simulink library "SimplusGT"  (R2018b)
settings: Solver=ode45  StartTime=0.0  StopTime=10.0  RelTol=1e-3
undefined symbols (not defined in the file): ang_r, Cf, DiscIntNeverNeededParam, initial, Lc, Lf, m, OtherInputs, P_dc, Sbase, t0, Tm_pu, Ts, V, Vbase, w_droop, w_i, w_pll, w_tau, w_v, Wbase, wc, wfil, x0, Ybase, Zbase
libraries: powerlib x334, SimplexPS_2015a x6, $bdroot x1
(part 3 of 8)

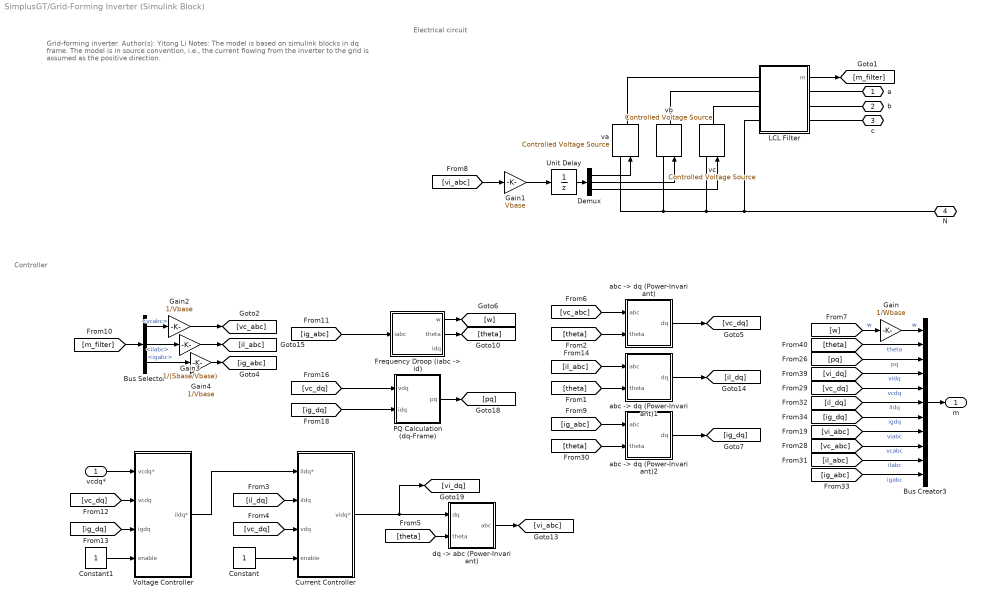
== system SimplusGT/Grid-Forming Inverter (Simulink Block) ==
  note: Controller
  note: Electrical circuit
  note: Grid-forming inverter.
      |
      | Author(s): Yitong Li
      |
      | Notes:
      |
      | The model is based on simulink blocks in dq frame.
      |
      | The model is in source convention, i.e., the current flowing from the inverter to the grid is assumed as the positive direction.
  vcdq* : Inport
  Bus Creator3 : BusCreator  Inputs=11
  Bus Selector : BusSelector  OutputSignals=vcabc,ilabc,igabc
  Constant : Constant
  Constant1 : Constant
  Current Controller : Subsystem  mask{Ts=Ts, Wbase=Wbase, Lf=Lf*(Vbase^2/Sbase)/Wbase, Kg=0, Kp=w_i*Lf*(Vbase^2/Sbase)/Wbase, Ki=w_i*w_i/4*Lf*(Vbase^2/Sbase)/Wbase, xdmax=inf, xqmax=inf, Kcd=0}
      mask prompts: Ts "Sampling Time (s)"; Wbase "Base Angular Frequency (rad/s)"; Lf "Inductance"; Kg "Estimator Gain"; Kp "Proportional Gain"; Ki "Integral Gain"; xdmax "Voltage D Limit"; xqmax "Voltage Q Limit"; Kcd "Cross Decoupling Gain"
  Demux : Demux  Outputs=3
  "Frequency Droop (iabc -> id)" : Subsystem  AncestorBlock=|  mask{Ts=Ts, Sbase=Sbase, Vbase=Vbase, Wbase=Wbase, m=m, w_tau=w_droop, theta0=0, i0=0, w0=1}
      | SimplusGT/Frequency Droop
      | (iabc -> id)
      mask prompts: Ts "Ts (s), samping period"; Sbase "Sbase (VA), base power"; Vbase "Vbase (V), base voltage"; Wbase "Wbase (rad/s), base angular frequency"; m "m (pu), droop gain"; w_tau "w_tau (rad/s), low-pass filter bandwidth"; theta0 "theta0 (rad), initial angle"; i0 "i0 (pu), current setting point"; w0 "w0 (pu), frequency setting point"
  Gain : Gain  Gain=1/Wbase
  Gain1 : Gain  Gain=Vbase
  Gain2 : Gain  Gain=1/Vbase
  Gain3 : Gain  Gain=1/(Sbase/Vbase)
  Gain4 : Gain  Gain=1/Vbase
  LCL Filter : Subsystem  AncestorBlock=SimplexPS/LCL Filter  mask{Lf=Lf*(Vbase^2/Sbase)/Wbase, Rf=1e-9, Lc=Lc*(Vbase^2/Sbase)/Wbase, Rc=1e-9, Cf=Cf*(Sbase/Vbase^2)/Wbase, Rd=1e-20}
      mask prompts: Lf "Lf (H)"; Rf "Rf (Ohm)"; Lc "Lc (H)"; Rc "Rc (Ohm)"; Cf "Cf (F)"; Rd "Rd (Ohm)"
  PQ Calculation (dq-Frame) : Subsystem  AncestorBlock=|
      | SimplusGT/PQ Calculation
      | (dq-Frame)
  Unit Delay : UnitDelay  SampleTime=-1
  Voltage Controller : Subsystem  mask{Ts=Ts, Wbase=Wbase, Cf=Cf*(Sbase/Vbase^2)/Wbase, Kg=0, Kp=w_v*Cf*(Sbase/Vbase^2)/Wbase, Ki=w_v*w_v/4*Cf*(Sbase/Vbase^2)/Wbase*100, xdmax=inf, xqmax=inf, Kcd=0}
      mask prompts: Ts "Sampling Time (s)"; Wbase "Base Angular Frequency (rad/s)"; Cf "Capacitance"; Kg "Estimator Gain"; Kp "Proportional Gain"; Ki "Integral Gain"; xdmax "Current D Limit"; xqmax "Current Q Limit"; Kcd "Cross Decoupling Gain"
  "abc -> dq (Power-Invariant)" : Subsystem  AncestorBlock=|
      | SimplusGT/abc -> dq
      | (Power-Invariant)
  "abc -> dq (Power-Invariant)1" : Subsystem  AncestorBlock=|
      | SimplusGT/abc -> dq
      | (Power-Invariant)
  "abc -> dq (Power-Invariant)2" : Subsystem  AncestorBlock=|
      | SimplusGT/abc -> dq
      | (Power-Invariant)
  "dq -> abc (Power-Invariant)" : Subsystem  AncestorBlock=|
      | SimplusGT/dq -> abc
      | (Power-Invariant)
  va : powerlib/Electrical Sources/Controlled Voltage Source  Initialize=on  Source_Type=AC  Amplitude=0  Phase=0  Frequency=0  Measurements=None
  vb : powerlib/Electrical Sources/Controlled Voltage Source  Initialize=on  Source_Type=AC  Amplitude=0  Phase=0  Frequency=0  Measurements=None
  vc : powerlib/Electrical Sources/Controlled Voltage Source  Initialize=on  Source_Type=AC  Amplitude=0  Phase=0  Frequency=0  Measurements=None
  a : PMIOPort  Side=Right
  b : PMIOPort  Port=2  Side=Right
  c : PMIOPort  Port=3  Side=Right
  N : PMIOPort  Port=4  Side=Right
  m : Outport
  wires:
  "dq -> abc (Power-Invariant)"/1(abc) -> [vi_abc]
  Bus Creator3/1 -> m/1
  LCL Filter/1(m) -> [m_filter]
  Demux/1 -> va/1
  Demux/2 -> vb/1
  Demux/3 -> vc/1
  [theta] -> "abc -> dq (Power-Invariant)"/2(theta)
  [theta] -> "abc -> dq (Power-Invariant)1"/2(theta)
  [vc_abc] -> "abc -> dq (Power-Invariant)"/1(abc)
  [il_abc] -> "abc -> dq (Power-Invariant)1"/1(abc)
  [ig_abc] -> "abc -> dq (Power-Invariant)2"/1(abc)
  [theta] -> "abc -> dq (Power-Invariant)2"/2(theta)
  Bus Selector/3 -> Gain4/1  "<igabc>"
  Bus Selector/2 -> Gain3/1  "<ilabc>"
  "Frequency Droop (iabc -> id)"/2(theta) -> [theta]
  "Frequency Droop (iabc -> id)"/1(w) -> [w]
  Constant/1 -> Current Controller/4(enable)
  [vc_dq] -> Current Controller/3(vdq)
  Current Controller/1(vidq*) -> [vi_dq], "dq -> abc (Power-Invariant)"/1(dq)
  [theta] -> "dq -> abc (Power-Invariant)"/2(theta)
  [vc_dq] -> PQ Calculation (dq-Frame)/1(vdq)
  PQ Calculation (dq-Frame)/1(pq) -> [pq]
  [ig_dq] -> PQ Calculation (dq-Frame)/2(idq)
  [il_dq] -> Current Controller/2(iIdq)
  [ig_abc] -> "Frequency Droop (iabc -> id)"/1(iabc)
  "abc -> dq (Power-Invariant)"/1(dq) -> [vc_dq]
  "abc -> dq (Power-Invariant)2"/1(dq) -> [ig_dq]
  "abc -> dq (Power-Invariant)1"/1(dq) -> [il_dq]
  [m_filter] -> Bus Selector/1
  Unit Delay/1 -> Demux/1
  Bus Selector/1 -> Gain2/1  "<vcabc>"
  [w] -> Gain/1  "w"
  Gain/1 -> Bus Creator3/1  "w"
  [theta] -> Bus Creator3/2  "theta"
  [pq] -> Bus Creator3/3  "pq"
  [vi_dq] -> Bus Creator3/4  "vidq"
  [vc_dq] -> Bus Creator3/5  "vcdq"
  [il_dq] -> Bus Creator3/6  "ildq"
  [ig_dq] -> Bus Creator3/7  "igdq"
  [vi_abc] -> Bus Creator3/8  "viabc"
  [vc_abc] -> Bus Creator3/9  "vcabc"
  [il_abc] -> Bus Creator3/10  "ilabc"
  [ig_abc] -> Bus Creator3/11  "igabc"
  vcdq*/1 -> Voltage Controller/1(vcdq*)
  Voltage Controller/1(ildq*) -> Current Controller/1(iIdq*)
  Constant1/1 -> Voltage Controller/4(enable)
  [vc_dq] -> Voltage Controller/2(vcdq)
  [ig_dq] -> Voltage Controller/3(igdq)
  Gain2/1 -> [vc_abc]
  Gain3/1 -> [il_abc]
  Gain4/1 -> [ig_abc]
  [vi_abc] -> Gain1/1
  Gain1/1 -> Unit Delay/1
  connections:
  LCL Filter/LConn2 -- vb/RConn1
  LCL Filter/LConn1 -- va/RConn1
  LCL Filter/RConn1 -- a/RConn1
  LCL Filter/RConn2 -- b/RConn1
  LCL Filter/RConn3 -- c/RConn1
  N/RConn1 -- LCL Filter/LConn4 -- vc/LConn1 -- vb/LConn1 -- va/LConn1
  LCL Filter/LConn3 -- vc/RConn1

== system SimplusGT/Hold ==
  note: Hold
      |
      | Author(s): Yitong Li
      |
      | Notes:
      |
      | This block can hold the input value to constant when "enable" is set from zero to one.
  In : Inport
  Enable : Inport  Port=2
  Memory : Memory
  Switch : Switch  Criteria=u2 > Threshold  Threshold=0.5
  Out : Outport
  wires:
  Switch/1 -> Memory/1, Out/1
  Enable/1 -> Switch/2
  Memory/1 -> Switch/1
  In/1 -> Switch/3

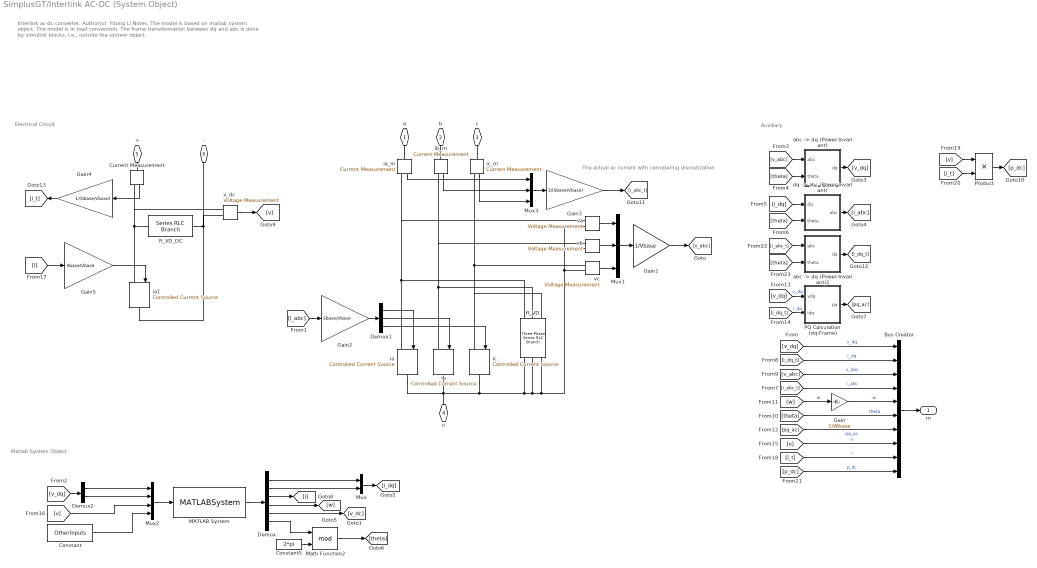
== system SimplusGT/Interlink AC-DC (System Object) ==
  note: Matlab System Object
  note: Auxiliary
  note: Electrical Circuit
  note: Interlink ac-dc converter.
      |
      | Author(s): Yitong Li
      |
      | Notes:
      |
      | The model is based on matlab system object.
      |
      | The model is in load convention.
      |
      | The frame transformation between dq and abc is done by simulink blocks, i.e., outside the system object.
  note: The actual ac current with considering discretization
  Bus Creator : BusCreator  Inputs=10
  Constant : Constant  Value=OtherInputs
  Constant5 : Constant  Value=2*pi
  Current Measurement : powerlib/Measurements/Current Measurement  PhasorSimulation=off  OutputType=Complex  PSBequivalent=0
  Demux : Demux  Outputs=6
  Demux1 : Demux  Outputs=3
  Demux2 : Demux  Outputs=2
  Gain : Gain  Gain=1/Wbase
  Gain1 : Gain  Gain=1/Vbase
  Gain2 : Gain  Gain=Sbase/Vbase
  Gain3 : Gain  Gain=1/(Sbase/Vbase)
  Gain4 : Gain  Gain=1/(Sbase/Vbase)
  Gain5 : Gain  Gain=Sbase/Vbase
  MATLAB System : MATLABSystem  System=SimplusGT.Class.InterlinkAcDc  Ts=Ts  Para=ApparatusPara  ApparatusType=ApparatusType  PowerFlow=PowerFlow  x0=x0  DiscreMethod=DiscreMethod  LinearizationTimes=LinearizationTimes  DirectFeedthrough=DirectFeedthrough  VirtualResistor=DiscreDampingFlag  EquiInitial=true  ElecPortIOs=[ 1, 2, 3 ]  SimulateUsing=Code generation
      mask Type: SimplusGT.Class.InterlinkAcDc
      mask Display:
      | disp('InterlinkAcDc');
      | port_label('input',1,'u');
      | port_label('output',1,'y');
  Math Function2 : Math  Operator=mod  SaturateOnIntegerOverflow=on
  Mux : Mux  Inputs=2
  Mux1 : Mux  Inputs=3
  Mux2 : Mux
  Mux3 : Mux  Inputs=3
  PQ Calculation (dq-Frame) : Subsystem  AncestorBlock=|
      | SimplusGT/PQ Calculation
      | (dq-Frame)
  Product : Product
  R_VD : powerlib/Elements/Three-Phase Series RLC Branch  LConnTagsString=A|B|C  RConnTagsString=A|B|C  BranchType=R  Resistance=DiscreDampingValue*Vbase^2/Sbase  Inductance=1e-3  Capacitance=1e-6  Measurements=None
  R_VD_DC : powerlib/Elements/Series RLC Branch  LConnTagsString=__new0  RConnTagsString=__new0  BranchType=R  Resistance=DiscreDampingValue*Vbase^2/Sbase  Inductance=1e-3  SetiL0=off  InitialCurrent=0  Capacitance=1e-6  Setx0=off  InitialVoltage=0  Measurements=None
  "abc -> dq (Power-Invariant)" : Subsystem  AncestorBlock=|
      | SimplusGT/abc -> dq
      | (Power-Invariant)
  "abc -> dq (Power-Invariant)1" : Subsystem  AncestorBlock=|
      | SimplusGT/abc -> dq
      | (Power-Invariant)
  "dq -> abc (Power-Invariant)" : Subsystem  AncestorBlock=|
      | SimplusGT/dq -> abc
      | (Power-Invariant)
  ia : powerlib/Electrical Sources/Controlled Current Source  Initialize=on  Source_Type=AC  Amplitude=0  Phase=0  Frequency=0  Measurements=None
  ia1 : powerlib/Electrical Sources/Controlled Current Source  Initialize=on  Source_Type=AC  Amplitude=0  Phase=0  Frequency=0  Measurements=None
  ia_m : powerlib/Measurements/Current Measurement  PhasorSimulation=off  OutputType=Complex  PSBequivalent=0
  ib : powerlib/Electrical Sources/Controlled Current Source  Initialize=on  Source_Type=AC  Amplitude=0  Phase=0  Frequency=0  Measurements=None
  ib_m : powerlib/Measurements/Current Measurement  PhasorSimulation=off  OutputType=Complex  PSBequivalent=0
  ic : powerlib/Electrical Sources/Controlled Current Source  Initialize=on  Source_Type=AC  Amplitude=0  Phase=0  Frequency=0  Measurements=None
  ic_m : powerlib/Measurements/Current Measurement  PhasorSimulation=off  OutputType=Complex  PSBequivalent=0
  v_dc : powerlib/Measurements/Voltage Measurement  PhasorSimulation=off  OutputType=Complex  PSBequivalent=0
  va : powerlib/Measurements/Voltage Measurement  PhasorSimulation=off  OutputType=Complex  PSBequivalent=0
  vb : powerlib/Measurements/Voltage Measurement  PhasorSimulation=off  OutputType=Complex  PSBequivalent=0
  vc : powerlib/Measurements/Voltage Measurement  PhasorSimulation=off  OutputType=Complex  PSBequivalent=0
  a : PMIOPort  Side=Left
  b : PMIOPort  Port=2  Side=Left
  c : PMIOPort  Port=3  Side=Left
  n : PMIOPort  Port=4  Side=Left
  + : PMIOPort  Port=5  Side=Left
  - : PMIOPort  Port=6  Side=Left
  m : Outport
  wires:
  Demux/2 -> Mux/2
  Demux/1 -> Mux/1
  Mux/1 -> [i_dq]
  Demux1/1 -> ia/1
  Demux1/2 -> ib/1
  va/1 -> Mux1/1
  vb/1 -> Mux1/2
  Mux1/1 -> Gain1/1
  [v_dq] -> Demux2/1
  Demux2/1 -> Mux2/1
  Demux2/2 -> Mux2/2
  [v_dq] -> Bus Creator/1  "v_dq"
  [i_dq_t] -> Bus Creator/2  "i_dq"
  [v_abc] -> Bus Creator/3  "v_abc"
  [i_abc_t] -> Bus Creator/4  "i_abc"
  [theta] -> Bus Creator/6  "theta"
  [v_abc] -> "abc -> dq (Power-Invariant)"/1(abc)
  [theta] -> "abc -> dq (Power-Invariant)"/2(theta)
  "abc -> dq (Power-Invariant)"/1(dq) -> [v_dq]
  [i_dq] -> "dq -> abc (Power-Invariant)"/1(dq)
  [theta] -> "dq -> abc (Power-Invariant)"/2(theta)
  "dq -> abc (Power-Invariant)"/1(abc) -> [i_abc]
  Mux2/1 -> MATLAB System/1
  MATLAB System/1 -> Demux/1
  vc/1 -> Mux1/3
  Demux1/3 -> ic/1
  Constant5/1 -> Math Function2/2
  Math Function2/1 -> [theta]
  Bus Creator/1 -> m/1
  Constant/1 -> Mux2/4
  [w] -> Gain/1  "w"
  Gain/1 -> Bus Creator/5  "w"
  [i_abc] -> Gain2/1
  [pq_ac] -> Bus Creator/7  "pq_ac"
  [v_dq] -> PQ Calculation (dq-Frame)/1(vdq)  "v_dq"
  [i_dq_t] -> PQ Calculation (dq-Frame)/2(idq)  "i_dq"
  PQ Calculation (dq-Frame)/1(pq) -> [pq_ac]
  Gain2/1 -> Demux1/1
  Gain1/1 -> [v_abc]
  [v] -> Bus Creator/8  "v"
  Demux/4 -> [w]
  Demux/5 -> [v_dc]
  Demux/6 -> Math Function2/1
  [v] -> Mux2/3
  Demux/3 -> [i]
  v_dc/1 -> [v]
  [i_t] -> Bus Creator/9  "i"
  [v] -> Product/1
  [i_t] -> Product/2
  Product/1 -> [p_dc]
  [p_dc] -> Bus Creator/10  "p_dc"
  ic_m/1 -> Mux3/3
  ib_m/1 -> Mux3/2
  Gain3/1 -> [i_abc_t]
  Mux3/1 -> Gain3/1
  ia_m/1 -> Mux3/1
  [theta] -> "abc -> dq (Power-Invariant)1"/2(theta)
  [i_abc_t] -> "abc -> dq (Power-Invariant)1"/1(abc)
  "abc -> dq (Power-Invariant)1"/1(dq) -> [i_dq_t]
  Gain4/1 -> [i_t]
  Current Measurement/1 -> Gain4/1
  [i] -> Gain5/1
  Gain5/1 -> ia1/1
  connections:
  vb/LConn2 -- va/LConn2 -- vc/LConn2 -- R_VD/RConn3 -- R_VD/RConn2 -- R_VD/RConn1 -- ic/RConn1 -- ia/RConn1 -- ib/RConn1 -- n/RConn1
  R_VD/LConn1 -- ia_m/RConn1 -- va/LConn1 -- ia/LConn1
  R_VD/LConn2 -- ib_m/RConn1 -- vb/LConn1 -- ib/LConn1
  R_VD/LConn3 -- ic/LConn1 -- ic_m/RConn1 -- vc/LConn1
  ia1/LConn1 -- Current Measurement/RConn1 -- v_dc/LConn1 -- R_VD_DC/LConn1
  ia1/RConn1 -- R_VD_DC/RConn1 -- -/RConn1 -- v_dc/LConn2
  c/RConn1 -- ic_m/LConn1
  b/RConn1 -- ib_m/LConn1
  a/RConn1 -- ia_m/LConn1
  Current Measurement/LConn1 -- +/RConn1

== system SimplusGT/L Filter (3ph) ==
  note: Model for a L filter.
      |
      | Author(s): Yitong Li
      |
      | Notes:
      |
      | vi is the converter side voltage, and vg is the grid side voltage.
  Bus Creator : BusCreator  Inputs=3
  "LL -> LN" : Subsystem  AncestorBlock=SimplusGT/LL -> LN
  "LL -> LN1" : Subsystem  AncestorBlock=SimplusGT/LL -> LN
  Mux : Mux  Inputs=3
  Mux1 : Mux  Inputs=3
  Mux2 : Mux  Inputs=3
  Three-Phase Series RLC Branch : powerlib/Elements/Three-Phase Series RLC Branch  LConnTagsString=A|B|C  RConnTagsString=A|B|C  BranchType=RL  Resistance=Rf  Inductance=Lf  Capacitance=1e-6  Measurements=None
  Vab : powerlib/Measurements/Voltage Measurement  PhasorSimulation=off  OutputType=Complex  PSBequivalent=0
  Vab1 : powerlib/Measurements/Voltage Measurement  PhasorSimulation=off  OutputType=Complex  PSBequivalent=0
  Vbc : powerlib/Measurements/Voltage Measurement  PhasorSimulation=off  OutputType=Complex  PSBequivalent=0
  Vbc1 : powerlib/Measurements/Voltage Measurement  PhasorSimulation=off  OutputType=Complex  PSBequivalent=0
  Vca : powerlib/Measurements/Voltage Measurement  PhasorSimulation=off  OutputType=Complex  PSBequivalent=0
  Vca1 : powerlib/Measurements/Voltage Measurement  PhasorSimulation=off  OutputType=Complex  PSBequivalent=0
  ila : powerlib/Measurements/Current Measurement  PhasorSimulation=off  OutputType=Complex  PSBequivalent=0
  ilb : powerlib/Measurements/Current Measurement  PhasorSimulation=off  OutputType=Complex  PSBequivalent=0
  ilc : powerlib/Measurements/Current Measurement  PhasorSimulation=off  OutputType=Complex  PSBequivalent=0
  via : PMIOPort  Side=Left
  vib : PMIOPort  Port=2  Side=Left
  vic : PMIOPort  Port=3  Side=Left
  vga : PMIOPort  Port=4  Side=Right
  vgb : PMIOPort  Port=5  Side=Right
  vgc : PMIOPort  Port=6  Side=Right
  m : Outport
  wires:
  Vab/1 -> Mux/1
  Vbc/1 -> Mux/2
  ilb/1 -> Mux2/2
  Vca/1 -> Mux/3
  Vca1/1 -> Mux1/3
  "LL -> LN1"/1(Out1) -> [vgabc]
  ilc/1 -> Mux2/3
  "LL -> LN"/1(Out1) -> [viabc]
  Mux1/1 -> "LL -> LN"/1(In1)
  Mux/1 -> "LL -> LN1"/1(In1)
  Vab1/1 -> Mux1/1
  ila/1 -> Mux2/1
  Mux2/1 -> [ilabc]
  Vbc1/1 -> Mux1/2
  [viabc] -> Bus Creator/1  "viabc"
  Bus Creator/1 -> m/1
  [vgabc] -> Bus Creator/2  "vgabc"
  [ilabc] -> Bus Creator/3  "ilabc"
  connections:
  Vca/LConn1 -- Vbc/LConn2 -- ilc/RConn1 -- vgc/RConn1
  Three-Phase Series RLC Branch/LConn1 -- via/RConn1 -- Vab1/LConn1 -- Vca1/LConn2
  Three-Phase Series RLC Branch/RConn2 -- ilb/LConn1
  Three-Phase Series RLC Branch/RConn3 -- ilc/LConn1
  Vab/LConn2 -- Vbc/LConn1 -- vgb/RConn1 -- ilb/RConn1
  Vbc1/LConn2 -- vic/RConn1 -- Three-Phase Series RLC Branch/LConn3 -- Vca1/LConn1
  Vab1/LConn2 -- vib/RConn1 -- Three-Phase Series RLC Branch/LConn2 -- Vbc1/LConn1
  Vca/LConn2 -- Vab/LConn1 -- ila/RConn1 -- vga/RConn1
  Three-Phase Series RLC Branch/RConn1 -- ila/LConn1

== system SimplusGT/LC Filter (3ph) ==
  note: Model for a LC filter.
      |
      | Author(s): Yitong Li
      |
      | Notes:
      |
      | vi is the converter side voltage, and vg is the grid side voltage.
  Bus Creator : BusCreator  Inputs=4
  "LL -> LN" : Subsystem  AncestorBlock=SimplusGT/LL -> LN
  Mux{1..4} (4 alike) : Mux  Inputs=3
  Three-Phase Series RLC Branch : powerlib/Elements/Three-Phase Series RLC Branch  LConnTagsString=A|B|C  RConnTagsString=A|B|C  BranchType=RL  Resistance=Rf  Inductance=Lf  Capacitance=1e-6  Measurements=None
  Three-Phase Series RLC Branch2 : powerlib/Elements/Three-Phase Series RLC Branch  LConnTagsString=A|B|C  RConnTagsString=A|B|C  BranchType=RC  Resistance=Rd  Inductance=Lc  Capacitance=Cf  Measurements=None
  Vab1 : powerlib/Measurements/Voltage Measurement  PhasorSimulation=off  OutputType=Complex  PSBequivalent=0
  Vbc1 : powerlib/Measurements/Voltage Measurement  PhasorSimulation=off  OutputType=Complex  PSBequivalent=0
  Vca1 : powerlib/Measurements/Voltage Measurement  PhasorSimulation=off  OutputType=Complex  PSBequivalent=0
  iga : powerlib/Measurements/Current Measurement  PhasorSimulation=off  OutputType=Complex  PSBequivalent=0
  igb : powerlib/Measurements/Current Measurement  PhasorSimulation=off  OutputType=Complex  PSBequivalent=0
  igc : powerlib/Measurements/Current Measurement  PhasorSimulation=off  OutputType=Complex  PSBequivalent=0
  ila : powerlib/Measurements/Current Measurement  PhasorSimulation=off  OutputType=Complex  PSBequivalent=0
  ilb : powerlib/Measurements/Current Measurement  PhasorSimulation=off  OutputType=Complex  PSBequivalent=0
  ilc : powerlib/Measurements/Current Measurement  PhasorSimulation=off  OutputType=Complex  PSBequivalent=0
  vca measure : powerlib/Measurements/Voltage Measurement  PhasorSimulation=off  OutputType=Complex  PSBequivalent=0
  vcb measure : powerlib/Measurements/Voltage Measurement  PhasorSimulation=off  OutputType=Complex  PSBequivalent=0
  vcc measure : powerlib/Measurements/Voltage Measurement  PhasorSimulation=off  OutputType=Complex  PSBequivalent=0
  via : PMIOPort  Side=Left
  vib : PMIOPort  Port=2  Side=Left
  vic : PMIOPort  Port=3  Side=Left
  vga : PMIOPort  Port=4  Side=Right
  vgb : PMIOPort  Port=5  Side=Right
  vgc : PMIOPort  Port=6  Side=Right
  N : PMIOPort  Port=7  Side=Left
  m : Outport
  wires:
  igb/1 -> Mux4/2
  iga/1 -> Mux4/1
  Vab1/1 -> Mux1/1
  vcb measure/1 -> Mux3/2
  [viabc] -> Bus Creator/1  "viabc"
  ilc/1 -> Mux2/3
  igc/1 -> Mux4/3
  ila/1 -> Mux2/1
  Mux1/1 -> "LL -> LN"/1(In1)
  Bus Creator/1 -> m/1
  vcc measure/1 -> Mux3/3
  ilb/1 -> Mux2/2
  vca measure/1 -> Mux3/1
  Mux3/1 -> [vcabc]
  "LL -> LN"/1(Out1) -> [viabc]
  Vca1/1 -> Mux1/3
  [vcabc] -> Bus Creator/2  "vcabc"
  Mux2/1 -> [ilabc]
  Mux4/1 -> [igabc]
  Vbc1/1 -> Mux1/2
  [ilabc] -> Bus Creator/3  "ilabc"
  [igabc] -> Bus Creator/4  "igabc"
  connections:
  Three-Phase Series RLC Branch2/LConn3 -- igc/LConn1 -- ilc/RConn1 -- vcc measure/LConn1
  Vbc1/LConn2 -- vic/RConn1 -- Three-Phase Series RLC Branch/LConn3 -- Vca1/LConn1
  Three-Phase Series RLC Branch/RConn3 -- ilc/LConn1
  vca measure/LConn1 -- ila/RConn1 -- iga/LConn1 -- Three-Phase Series RLC Branch2/LConn1
  vga/RConn1 -- iga/RConn1
  vgb/RConn1 -- igb/RConn1
  vcb measure/LConn1 -- igb/LConn1 -- ilb/RConn1 -- Three-Phase Series RLC Branch2/LConn2
  Vab1/LConn2 -- vib/RConn1 -- Three-Phase Series RLC Branch/LConn2 -- Vbc1/LConn1
  vgc/RConn1 -- igc/RConn1
  vcc measure/LConn2 -- vca measure/LConn2 -- vcb measure/LConn2 -- N/RConn1 -- Three-Phase Series RLC Branch2/RConn1 -- Three-Phase Series RLC Branch2/RConn2 -- Three-Phase Series RLC Branch2/RConn3
  Three-Phase Series RLC Branch/LConn1 -- via/RConn1 -- Vab1/LConn1 -- Vca1/LConn2
  Three-Phase Series RLC Branch/RConn1 -- ila/LConn1
  Three-Phase Series RLC Branch/RConn2 -- ilb/LConn1

== system SimplusGT/LCL Filter (3ph) ==
  note: Model for a LCL filter.
      |
      | Author(s): Yitong Li
      |
      | Notes:
      |
      | vi is the converter side voltage, and vg is the grid side voltage.
  Bus Creator : BusCreator  Inputs=5
  "LL -> LN" : SimplexPS_2015a/LL -> LN  SystemSampleTime=-1
      settings: SourceProductName=Some kind of I/O error occurred when accessing database \\icnas1.cc.ic.ac.uk\yz34218\appdata\MathWorks\MATLAB\R2018b\slblocks_master.db. (disk I/O error)
  "LL -> LN1" : SimplexPS_2015a/LL -> LN  SystemSampleTime=-1
      settings: SourceProductName=Some kind of I/O error occurred when accessing database \\icnas1.cc.ic.ac.uk\yz34218\appdata\MathWorks\MATLAB\R2018b\slblocks_master.db. (disk I/O error)
  Mux{,1..4} (5 alike) : Mux  Inputs=3
  Three-Phase Series RLC Branch : powerlib/Elements/Three-Phase Series RLC Branch  LConnTagsString=A|B|C  RConnTagsString=A|B|C  BranchType=RL  Resistance=Rf  Inductance=Lf  Capacitance=1e-6  Measurements=None
  Three-Phase Series RLC Branch1 : powerlib/Elements/Three-Phase Series RLC Branch  LConnTagsString=A|B|C  RConnTagsString=A|B|C  BranchType=RL  Resistance=Rc  Inductance=Lc  Capacitance=1e-6  Measurements=None
  Three-Phase Series RLC Branch2 : powerlib/Elements/Three-Phase Series RLC Branch  LConnTagsString=A|B|C  RConnTagsString=A|B|C  BranchType=RC  Resistance=Rd  Inductance=Lc  Capacitance=Cf  Measurements=None
  Vab : powerlib/Measurements/Voltage Measurement  PhasorSimulation=off  OutputType=Complex  PSBequivalent=0
  Vab1 : powerlib/Measurements/Voltage Measurement  PhasorSimulation=off  OutputType=Complex  PSBequivalent=0
  Vbc : powerlib/Measurements/Voltage Measurement  PhasorSimulation=off  OutputType=Complex  PSBequivalent=0
  Vbc1 : powerlib/Measurements/Voltage Measurement  PhasorSimulation=off  OutputType=Complex  PSBequivalent=0
  Vca : powerlib/Measurements/Voltage Measurement  PhasorSimulation=off  OutputType=Complex  PSBequivalent=0
  Vca1 : powerlib/Measurements/Voltage Measurement  PhasorSimulation=off  OutputType=Complex  PSBequivalent=0
  iga : powerlib/Measurements/Current Measurement  PhasorSimulation=off  OutputType=Complex  PSBequivalent=0
  igb : powerlib/Measurements/Current Measurement  PhasorSimulation=off  OutputType=Complex  PSBequivalent=0
  igc : powerlib/Measurements/Current Measurement  PhasorSimulation=off  OutputType=Complex  PSBequivalent=0
  ila : powerlib/Measurements/Current Measurement  PhasorSimulation=off  OutputType=Complex  PSBequivalent=0
  ilb : powerlib/Measurements/Current Measurement  PhasorSimulation=off  OutputType=Complex  PSBequivalent=0
  ilc : powerlib/Measurements/Current Measurement  PhasorSimulation=off  OutputType=Complex  PSBequivalent=0
  vca measure : powerlib/Measurements/Voltage Measurement  PhasorSimulation=off  OutputType=Complex  PSBequivalent=0
  vcb measure : powerlib/Measurements/Voltage Measurement  PhasorSimulation=off  OutputType=Complex  PSBequivalent=0
  vcc measure : powerlib/Measurements/Voltage Measurement  PhasorSimulation=off  OutputType=Complex  PSBequivalent=0
  via : PMIOPort  Side=Left
  vib : PMIOPort  Port=2  Side=Left
  vic : PMIOPort  Port=3  Side=Left
  vga : PMIOPort  Port=4  Side=Right
  vgb : PMIOPort  Port=5  Side=Right
  vgc : PMIOPort  Port=6  Side=Right
  N : PMIOPort  Port=7  Side=Left
  m : Outport
  wires:
  Mux4/1 -> [igabc]
  ilb/1 -> Mux2/2
  ila/1 -> Mux2/1
  igc/1 -> Mux4/3
  vcc measure/1 -> Mux3/3
  Vab/1 -> Mux/1
  Mux/1 -> "LL -> LN1"/1
  vca measure/1 -> Mux3/1
  vcb measure/1 -> Mux3/2
  igb/1 -> Mux4/2
  iga/1 -> Mux4/1
  Vca/1 -> Mux/3
  ilc/1 -> Mux2/3
  Vbc/1 -> Mux/2
  Mux2/1 -> [ilabc]
  Bus Creator/1 -> m/1
  "LL -> LN1"/1 -> [vgabc]
  Mux3/1 -> [vcabc]
  Vbc1/1 -> Mux1/2
  Vca1/1 -> Mux1/3
  Mux1/1 -> "LL -> LN"/1
  Vab1/1 -> Mux1/1
  "LL -> LN"/1 -> [viabc]
  [viabc] -> Bus Creator/1  "viabc"
  [vcabc] -> Bus Creator/2  "vcabc"
  [vgabc] -> Bus Creator/3  "vgabc"
  [ilabc] -> Bus Creator/4  "ilabc"
  [igabc] -> Bus Creator/5  "igabc"
  connections:
  vca measure/LConn2 -- Three-Phase Series RLC Branch2/RConn1 -- Three-Phase Series RLC Branch2/RConn2 -- N/RConn1 -- Three-Phase Series RLC Branch2/RConn3 -- vcc measure/LConn2 -- vcb measure/LConn2
  igc/RConn1 -- Vca/LConn1 -- Vbc/LConn2 -- vgc/RConn1
  Vbc1/LConn2 -- Three-Phase Series RLC Branch/LConn3 -- vic/RConn1 -- Vca1/LConn1
  Vab1/LConn2 -- vib/RConn1 -- Three-Phase Series RLC Branch/LConn2 -- Vbc1/LConn1
  Vca1/LConn2 -- Three-Phase Series RLC Branch/LConn1 -- via/RConn1 -- Vab1/LConn1
  ilc/RConn1 -- Three-Phase Series RLC Branch1/LConn3 -- vcc measure/LConn1 -- Three-Phase Series RLC Branch2/LConn3
  Three-Phase Series RLC Branch1/RConn2 -- igb/LConn1
  igb/RConn1 -- vgb/RConn1 -- Vbc/LConn1 -- Vab/LConn2
  vcb measure/LConn1 -- ilb/RConn1 -- Three-Phase Series RLC Branch1/LConn2 -- Three-Phase Series RLC Branch2/LConn2
  vca measure/LConn1 -- ila/RConn1 -- Three-Phase Series RLC Branch1/LConn1 -- Three-Phase Series RLC Branch2/LConn1
  Vca/LConn2 -- Vab/LConn1 -- vga/RConn1 -- iga/RConn1
  Three-Phase Series RLC Branch1/RConn1 -- iga/LConn1
  Three-Phase Series RLC Branch1/RConn3 -- igc/LConn1
  Three-Phase Series RLC Branch/RConn1 -- ila/LConn1
  Three-Phase Series RLC Branch/RConn2 -- ilb/LConn1
  Three-Phase Series RLC Branch/RConn3 -- ilc/LConn1

== system SimplusGT/LL -> LN ==
  note: Transformation from line-to-line voltage to line-to-neutral voltage.
      |
      | Author(s): Yitong Li
  In1 : Inport
  Fcn : Fcn  Expr=u[1]-u[3]
  Fcn1 : Fcn  Expr=u[2]-u[1]
  Fcn2 : Fcn  Expr=u[3]-u[2]
  Gain : Gain  Gain=1/3
  Mux9 : Mux  Inputs=3
  Out1 : Outport
  wires:
  Fcn/1 -> Mux9/1
  Fcn1/1 -> Mux9/2
  Fcn2/1 -> Mux9/3
  Mux9/1 -> Out1/1
  Gain/1 -> Fcn2/1, Fcn1/1, Fcn/1
  In1/1 -> Gain/1

== system SimplusGT/Load Impulse ==
  note: Model for an impulse load.
      |
      | Author(s): Yitong Li
  Single Pulse : $bdroot/Single Pulse  t0=t0  dt=dt  Am=1
  Three-Phase Breaker : powerlib/Elements/Three-Phase Breaker  InitialState=open  SwitchA=on  SwitchB=on  SwitchC=on  SwitchTimes="[1/60  5/60]"  External=on  BreakerResistance=0.01  SnubberResistance=1e6  SnubberCapacitance=inf  Measurements=None
  load : powerlib/Elements/Three-Phase Parallel RLC Branch  LConnTagsString=A|B|C  RConnTagsString=A|B|C  BranchType=R  Resistance=R  Inductance=1  Capacitance=1  Measurements=None
      settings: SourceProductName=Simscape Power Systems  SourceProductBaseCode=PS
  a : PMIOPort  Side=Left
  b : PMIOPort  Port=2  Side=Left
  c : PMIOPort  Port=3  Side=Left
  n : PMIOPort  Port=4  Side=Right
  wires:
  Single Pulse/1 -> Three-Phase Breaker/1
  connections:
  load/RConn2 -- load/RConn3 -- load/RConn1 -- n/RConn1
  Three-Phase Breaker/RConn1 -- load/LConn3
  Three-Phase Breaker/RConn2 -- load/LConn2
  Three-Phase Breaker/RConn3 -- load/LConn1
  c/RConn1 -- Three-Phase Breaker/LConn1
  b/RConn1 -- Three-Phase Breaker/LConn2
  a/RConn1 -- Three-Phase Breaker/LConn3

== system SimplusGT/Load Step ==
  note: Model for a step load.
      |
      | Author(s): Yitong Li
  Constant : Constant  Value=Reverse
  Step : Step  Time=t0  SampleTime=0
  Step1 : Step  Time=t0  Before=1  After=0  SampleTime=0
  Switch : Switch  Criteria=u2 > Threshold  Threshold=0.5
  Three-Phase Breaker : powerlib/Elements/Three-Phase Breaker  InitialState=open  SwitchA=on  SwitchB=on  SwitchC=on  SwitchTimes="[1/60  5/60]"  External=on  BreakerResistance=0.01  SnubberResistance=1e6  SnubberCapacitance=inf  Measurements=None
  load : powerlib/Elements/Three-Phase Parallel RLC Branch  LConnTagsString=A|B|C  RConnTagsString=A|B|C  BranchType=R  Resistance=R  Inductance=1  Capacitance=1  Measurements=None
      settings: SourceProductName=Simscape Power Systems  SourceProductBaseCode=PS
  a : PMIOPort  Side=Left
  b : PMIOPort  Port=2  Side=Left
  c : PMIOPort  Port=3  Side=Left
  n : PMIOPort  Port=4  Side=Right
  wires:
  Switch/1 -> Three-Phase Breaker/1
  Constant/1 -> Switch/2
  Step1/1 -> Switch/1
  Step/1 -> Switch/3
  connections:
  a/RConn1 -- Three-Phase Breaker/LConn3
  b/RConn1 -- Three-Phase Breaker/LConn2
  Three-Phase Breaker/RConn3 -- load/LConn1
  Three-Phase Breaker/RConn2 -- load/LConn2
  load/RConn2 -- n/RConn1 -- load/RConn3 -- load/RConn1
  Three-Phase Breaker/RConn1 -- load/LConn3
  c/RConn1 -- Three-Phase Breaker/LConn1

== system SimplusGT/PLL (vDQ -> vq) ==
  note: Gpll
  note: Measurement
  note: Phase lock loop (PLL)
      |
      | Author(s): Yitong Li
      |
      | Notes:
      |
      | vq is fed into the PI controller of the PLL.
      |
      | This PLL assumes the input voltage is in DQ frame, which is the common electrical frame. It is not a practical PLL which uses vabc as the input. But this PLL is useful in research.
  vDQ : Inport
  wDQ : Inport  Port=2
  Constant1 : Constant
  Constant2 : Constant  Value=theta0
  Constant3 : Constant
  Constant4 : Constant  Value=2*pi
  Constant6 : Constant  Value=0
  Demux1 : Demux  Outputs=2
  Discrete PI1 : Subsystem  AncestorBlock=SimplusGT/Discrete PI  mask{Kp=w_pll, Ki=w_pll*w_pll/4, xmax=inf, xmin=-inf, Ts=Ts}
      mask prompts: Kp "Proportional Gain"; Ki "Integral Gain"; xmax "Upper Limit"; xmin "Lower Limit"; Ts "Sampling Time"
  Discrete-Time Integrator : DiscreteIntegrator  SampleTime=Ts  ICPrevOutput=DiscIntNeverNeededParam  ICPrevScaledInput=DiscIntNeverNeededParam
  Filter p : DiscreteTransferFcn  Numerator=w_tau*Ts  Denominator=[1 ((w_tau*Ts)-1)]  SampleTime=Ts
  Gain1 : Gain  Gain=Wbase
  Gain2 : Gain  Gain=1/Vbase
  Gain4 : Gain  Gain=1/Wbase
  Gain5 : Gain  Gain=1/pi
  Math Function1 : Math  Operator=mod  SaturateOnIntegerOverflow=on
  Mux : Mux  Inputs=2
  Scope : Scope  NumInputPorts=4
  Sum : Sum
  Sum1 : Sum
  Sum2 : Sum  Inputs=+-
  "x1y1 -> x2y2" : Subsystem  AncestorBlock=SimplusGT/x1y1 -> x2y2
  wdq : Outport
  theta : Outport  Port=2
  vdq : Outport  Port=3
  wires:
  [theta0] -> Mux/1  "theta0"
  Constant2/1 -> [theta0], Sum1/2
  Math Function1/1 -> "x1y1 -> x2y2"/2(theta), theta/1, [theta]
  Sum1/1 -> Math Function1/1
  Demux1/2 -> [vq], Gain2/1
  vDQ/1 -> "x1y1 -> x2y2"/1(x1y1)
  Discrete-Time Integrator/1 -> Sum1/1
  Gain2/1 -> Filter p/1
  [vd] -> Scope/1  "vd"
  Mux/1 -> Gain5/1
  Discrete PI1/1(Out) -> Sum/1
  "x1y1 -> x2y2"/1(x2y2) -> vdq/1, Demux1/1
  [w] -> Gain4/1  "w"
  Constant4/1 -> Math Function1/2
  [theta] -> Mux/2  "theta"
  Demux1/1 -> [vd]
  Gain5/1 -> Scope/4
  Constant1/1 -> Discrete PI1/1(enable)
  Gain4/1 -> Scope/3
  Gain1/1 -> Sum/2
  Constant3/1 -> Gain1/1
  [vq] -> Scope/2  "vq"
  Filter p/1 -> Discrete PI1/2(reference)
  Constant6/1 -> Discrete PI1/4(actual), Discrete PI1/3(initial)
  Sum/1 -> Sum2/1
  Sum2/1 -> [w], wdq/1, Discrete-Time Integrator/1
  wDQ/1 -> Sum2/2

== system SimplusGT/PLL (vabc -> theta) ==
  note: Measurement
  note: Gpll
  note: Phase lock loop (PLL)
      |
      | Author(s): Yitong Li
      |
      | Notes:
      |
      | theta of voltage is fed into the PI controller of the PLL.
  vabc : Inport
  Constant1 : Constant
  Constant2 : Constant  Value=2*pi
  Constant3 : Constant  Value=0
  Constant4 : Constant
  Constant5 : Constant  Value=theta0
  Demux : Demux  Outputs=2
  Discrete PI : Subsystem  AncestorBlock=SimplusGT/Discrete PI  mask{Kp=w_pll, Ki=w_pll*w_pll/4, xmax=inf, xmin=-inf, Ts=Ts}
      mask prompts: Kp "Proportional Gain"; Ki "Integral Gain"; xmax "Upper Limit"; xmin "Lower Limit"; Ts "Sampling Time"
  Discrete-Time Integrator : DiscreteIntegrator  SampleTime=Ts  ICPrevOutput=DiscIntNeverNeededParam  ICPrevScaledInput=DiscIntNeverNeededParam
  Filter p : DiscreteTransferFcn  Numerator=w_tau*Ts  Denominator=[1 ((w_tau*Ts)-1)]  SampleTime=Ts
  Gain1 : Gain  Gain=Wbase
  Gain4 : Gain  Gain=1/Wbase
  Gain5 : Gain  Gain=1/pi
  Math Function1 : Math  Operator=mod  SaturateOnIntegerOverflow=on
  Mux : Mux  Inputs=2
  Scope : Scope  NumInputPorts=4
  Selector : Selector  InputPortWidth=2  IndexOptions=Index vector (dialog)  Indices=[2 1]  OutputSizes=1
  Sum : Sum
  Sum1 : Sum
  Trigonometric Function : Trigonometry  Operator=atan2
  "abc -> dq (Power-Invariant)" : Subsystem  AncestorBlock=|
      | SimplusGT/abc -> dq
      | (Power-Invariant)
  w : Outport
  theta : Outport  Port=2
  vdq : Outport  Port=3
  wires:
  Constant2/1 -> Math Function1/2
  Constant1/1 -> Discrete PI/1(enable)
  Constant3/1 -> Discrete PI/3(initial), Discrete PI/4(actual)
  Trigonometric Function/1 -> Filter p/1
  Demux/1 -> [vq], Trigonometric Function/1
  Demux/2 -> [vd], Trigonometric Function/2
  Selector/1 -> Demux/1
  Math Function1/1 -> "abc -> dq (Power-Invariant)"/2(theta), [theta], theta/1
  "abc -> dq (Power-Invariant)"/1(dq) -> vdq/1, Selector/1
  vabc/1 -> "abc -> dq (Power-Invariant)"/1(abc)
  Discrete PI/1(Out) -> Sum/1
  Constant4/1 -> Gain1/1
  Sum/1 -> [w], w/1, Discrete-Time Integrator/1
  Filter p/1 -> Discrete PI/2(reference)
  [vq] -> Scope/2  "vq"
  Mux/1 -> Gain5/1
  [vd] -> Scope/1  "vd"
  [theta] -> Mux/2  "theta"
  Gain5/1 -> Scope/4
  Gain4/1 -> Scope/3
  [w] -> Gain4/1  "w"
  [theta0] -> Mux/1  "theta0"
  Gain1/1 -> Sum/2
  Discrete-Time Integrator/1 -> Sum1/1
  Sum1/1 -> Math Function1/1
  Constant5/1 -> [theta0], Sum1/2

== system SimplusGT/PLL (vabc -> vd+jvq) ==
  note: Measurement
  note: Frame trabsformation
  note: -j
  note: Gpll
  note: Gpll
  note: Phase lock loop (PLL)
      |
      | Author(s): Yitong Li
      |
      | Notes:
      |
      | This is a symmetric PLL controls both d- and q-axis voltage.
      |
      | It is built based on Dongsheng Yang's paper: "Symmetrical PLL for SISO Impedance Modeling and Enhanced Stability in Weak Grids", IEEE Transactions on Power Electronics, 2020.
  vabc : Inport
  Constant{,2..3,7} (4 alike) : Constant
  Constant{1,5..6,8} (4 alike) : Constant  Value=0
  Constant10 : Constant  Value=theta_d0
  Constant4 : Constant  Value=2*pi
  Constant9 : Constant  Value=theta_q0
  Demux1 : Demux  Outputs=2
  Discrete PI_d : Subsystem  AncestorBlock=SimplusGT/Discrete PI  mask{Kp=w_pll, Ki=w_pll*w_pll/4, xmax=inf, xmin=-inf, Ts=Ts}
      mask prompts: Kp "Proportional Gain"; Ki "Integral Gain"; xmax "Upper Limit"; xmin "Lower Limit"; Ts "Sampling Time"
  Discrete PI_q : Subsystem  AncestorBlock=SimplusGT/Discrete PI  mask{Kp=w_pll, Ki=w_pll*w_pll/4, xmax=inf, xmin=-inf, Ts=Ts}
      mask prompts: Kp "Proportional Gain"; Ki "Integral Gain"; xmax "Upper Limit"; xmin "Lower Limit"; Ts "Sampling Time"
  Discrete-Time Integrator : DiscreteIntegrator  SampleTime=Ts  ICPrevOutput=DiscIntNeverNeededParam  ICPrevScaledInput=DiscIntNeverNeededParam
  Discrete-Time Integrator1 : DiscreteIntegrator  SampleTime=Ts  ICPrevOutput=DiscIntNeverNeededParam  ICPrevScaledInput=DiscIntNeverNeededParam
  Exp : Math  SaturateOnIntegerOverflow=on
  Filter p : DiscreteTransferFcn  Numerator=w_tau*Ts  Denominator=[1 ((w_tau*Ts)-1)]  SampleTime=Ts
  Filter p1 : DiscreteTransferFcn  Numerator=w_tau*Ts  Denominator=[1 ((w_tau*Ts)-1)]  SampleTime=Ts
  Gain : Gain  Gain=Wbase
  Gain1 : Gain  Gain=Wbase
  Gain2 : Gain  Gain=1/Wbase
  Gain3 : Gain  Gain=-1
  Gain4 : Gain  Gain=1/pi
  Gain5 : Gain  Gain=1/Vbase
  Math Function1 : Math  Operator=mod  SaturateOnIntegerOverflow=on
  Mux : Mux  Inputs=2
  Mux1 : Mux  Inputs=2
  Mux2 : Mux  Inputs=2
  Product : Product
  Scope : Scope  NumInputPorts=3
  Sum : Sum  Inputs=|+-
  Sum{1..2,4..5} (4 alike) : Sum
  Sum3 : Sum  Inputs=|+-
  "abc -> dq (Power-Invariant)" : Subsystem  AncestorBlock=|
      | SimplusGT/abc -> dq
      | (Power-Invariant)
  wd : Outport
  theta_d : Outport  Port=2
  wq : Outport  Port=3
  theta_q : Outport  Port=4
  wires:
  Constant4/1 -> Math Function1/2
  Constant6/1 -> Discrete PI_q/3(initial), Discrete PI_q/4(actual)
  Demux1/2 -> [vq]
  Constant3/1 -> Discrete PI_q/1(enable)
  Math Function1/1 -> theta_d/1, [thetad]
  "abc -> dq (Power-Invariant)"/1(dq) -> Gain5/1
  Gain5/1 -> Demux1/1
  Demux1/1 -> [vd]
  Constant/1 -> Sum/2
  Sum/1 -> Discrete PI_d/2(reference)
  Constant7/1 -> Discrete PI_d/1(enable)
  Constant1/1 -> Discrete PI_d/4(actual), Discrete PI_d/3(initial)
  [thetad] -> "abc -> dq (Power-Invariant)"/2(theta)
  vabc/1 -> Product/1
  Product/1 -> "abc -> dq (Power-Invariant)"/1(abc)
  Exp/1 -> Product/2
  Gain3/1 -> theta_q/1, [thetaq]
  [vq] -> Filter p/1
  [vd] -> Filter p1/1
  Filter p1/1 -> Sum/1
  [thetaq] -> Exp/1
  Sum1/1 -> [wd], wd/1, Discrete-Time Integrator/1
  Discrete PI_q/1(Out) -> Sum1/1
  Sum2/1 -> Discrete-Time Integrator1/1, wq/1, [wq]
  Discrete PI_d/1(Out) -> Sum2/1
  Constant2/1 -> Gain/1
  Constant5/1 -> Gain1/1
  Filter p/1 -> Sum3/1
  Constant8/1 -> Sum3/2
  Sum3/1 -> Discrete PI_q/2(reference)
  Discrete-Time Integrator1/1 -> Sum4/1
  Sum4/1 -> Gain3/1
  Constant9/1 -> Sum4/2
  Gain/1 -> Sum1/2
  Gain1/1 -> Sum2/2
  Discrete-Time Integrator/1 -> Sum5/1
  Sum5/1 -> Math Function1/1
  Constant10/1 -> Sum5/2
  [vd] -> Mux/1
  [vq] -> Mux/2
  [wd] -> Mux1/1
  [wq] -> Mux1/2
  [thetad] -> Mux2/1
  [thetaq] -> Mux2/2
  Mux/1 -> Scope/1  "vdq"
  Mux1/1 -> Gain2/1  "wdq"
  Mux2/1 -> Gain4/1  "thetadq"
  Gain2/1 -> Scope/2
  Gain4/1 -> Scope/3

== system SimplusGT/PLL (vabc -> vq) ==
  note: Measurement
  note: Gpll
  note: Phase lock loop (PLL)
      |
      | Author(s): Yitong Li
      |
      | Notes:
      |
      | vq is fed into the PI controller of the PLL.
  vabc : Inport
  Constant1 : Constant
  Constant2 : Constant  Value=theta0
  Constant3 : Constant
  Constant4 : Constant  Value=2*pi
  Constant6 : Constant  Value=0
  Demux1 : Demux  Outputs=2
  Discrete PI : Subsystem  AncestorBlock=SimplusGT/Discrete PI  mask{Kp=w_pll, Ki=w_pll*w_pll/4, xmax=inf, xmin=-inf, Ts=Ts}
      mask prompts: Kp "Proportional Gain"; Ki "Integral Gain"; xmax "Upper Limit"; xmin "Lower Limit"; Ts "Sampling Time"
  Discrete-Time Integrator : DiscreteIntegrator  SampleTime=Ts  ICPrevOutput=DiscIntNeverNeededParam  ICPrevScaledInput=DiscIntNeverNeededParam
  Filter p : DiscreteTransferFcn  Numerator=w_tau*Ts  Denominator=[1 ((w_tau*Ts)-1)]  SampleTime=Ts
  Gain1 : Gain  Gain=Wbase
  Gain2 : Gain  Gain=1/Vbase
  Gain4 : Gain  Gain=1/Wbase
  Gain5 : Gain  Gain=1/pi
  Math Function1 : Math  Operator=mod  SaturateOnIntegerOverflow=on
  Mux : Mux  Inputs=2
  Scope : Scope  NumInputPorts=4
  Sum : Sum
  Sum1 : Sum
  "abc -> dq (Power-Invariant)" : Subsystem  AncestorBlock=|
      | SimplusGT/abc -> dq
      | (Power-Invariant)
  w : Outport
  theta : Outport  Port=2
  vdq : Outport  Port=3
  wires:
  vabc/1 -> "abc -> dq (Power-Invariant)"/1(abc)
  "abc -> dq (Power-Invariant)"/1(dq) -> vdq/1, Demux1/1
  Constant4/1 -> Math Function1/2
  Gain2/1 -> Filter p/1
  Demux1/2 -> [vq], Gain2/1
  Constant6/1 -> Discrete PI/4(actual), Discrete PI/3(initial)
  Constant1/1 -> Discrete PI/1(enable)
  Discrete PI/1(Out) -> Sum/1
  Sum/1 -> [w], w/1, Discrete-Time Integrator/1
  Gain1/1 -> Sum/2
  Discrete-Time Integrator/1 -> Sum1/1
  Sum1/1 -> Math Function1/1
  Constant2/1 -> [theta0], Sum1/2
  Filter p/1 -> Discrete PI/2(reference)
  [vq] -> Scope/2  "vq"
  Mux/1 -> Gain5/1
  Gain4/1 -> Scope/3
  [w] -> Gain4/1  "w"
  [theta0] -> Mux/1  "theta0"
  [vd] -> Scope/1  "vd"
  Gain5/1 -> Scope/4
  [theta] -> Mux/2  "theta"
  Demux1/1 -> [vd]
  Constant3/1 -> Gain1/1
  Math Function1/1 -> "abc -> dq (Power-Invariant)"/2(theta), [theta], theta/1

== system SimplusGT/PQ Calculation (dq-Frame) ==
  note: Power calculation.
      |
      | Author(s): Yitong Li
      |
      | Notes:
      |
      | The calculation is done in dq frame.
  vdq : Inport
  idq : Inport  Port=2
  Mux : Mux  Inputs=2
  Mux1 : Mux  Inputs=2
  P = vd*id+vq*iq : Fcn  Expr=u[1]*u[3]+u[2]*u[4]
  Q = -vd*iq+vq*id : Fcn  Expr=-u[1]*u[4]+u[2]*u[3]
  pq : Outport
  wires:
  Q = -vd*iq+vq*id/1 -> Mux/2
  Mux1/1 -> Q = -vd*iq+vq*id/1, P = vd*id+vq*iq/1
  idq/1 -> Mux1/2
  vdq/1 -> Mux1/1
  P = vd*id+vq*iq/1 -> Mux/1
  Mux/1 -> pq/1

== system SimplusGT/ReIm2Complex ==
  note: Transformation from real/imaginary to complex vectors
      |
      | Author(s): Yitong Li
      |
      | Notes:
      |
      | A example is from dq frame to dq+- frame.
  Re Im : Inport
  -> backward : Fcn  Expr=u[1] - u[2]*1i
  -> forward : Fcn  Expr=u[1] + u[2]*1i
  Mux : Mux  Inputs=2
  +- : Outport
  wires:
  Re Im/1 -> -> backward/1, -> forward/1
  Mux/1 -> +-/1
  -> forward/1 -> Mux/1
  -> backward/1 -> Mux/2

== system SimplusGT/Recycle Bin ==
  Synchronous Machine (dq-Frame System Object) (Internal Frame Transformation) : Subsystem  mask{Ts=Ts, Sbase=Sbase, Vbase=Vbase, Wbase=Wbase, DeviceType=0, DevicePara=[], PowerFlow=[], x0=[0;0;Wbase;0], OtherInputs=[Tm_pu/Wbase;0], DiscreMethod=Hybrid Trapezoidal, EnableInsideModification=off, DiscreDampingFlag=on, DiscreDampingValue=0, LinearizationTimes=1, DirectFeedthrough=off}
      mask prompts: Ts "Ts (s), samping period"; Sbase "Sbase (VA), power base"; Vbase "Vbase (V), voltage base"; Wbase "Wbase (rad/s), frequency base"; DeviceType "Device type"; DevicePara "Device parameters"; PowerFlow "Power flow paramters"; x0 "x0, initial states"; OtherInputs "Other inputs"; DiscreMethod "Discrerization method"; EnableInsideModification "Enable inside modification"; DiscreDampingFlag "Enable discretization damping"; DiscreDampingValue "Discretization damping value"; LinearizationTimes "Linearization times"; DirectFeedthrough "Direct feedthrough"
      mask init:
      | SimplexPS.Simulink.DeviceMaskInitialization(EnableInsideModification,DiscreDampingFlag);
      mask TypeOptions DiscreMethod: Forward Euler | Hybrid Trapezoidal | Virtual Damping
      mask TypeOptions LinearizationTimes: 1 | 2

== system SimplusGT/Root Mean Squre ==
  note: Root mean squre
      |
      | Author(s): Yitong Li
  x : Inport
  y : Inport  Port=2
  Math Function1 : Math  Operator=square  SaturateOnIntegerOverflow=on
  Math Function2 : Math  Operator=square  SaturateOnIntegerOverflow=on
  Sqrt : Sqrt  SaturateOnIntegerOverflow=on
  Sum : Sum
  RMS : Outport
  wires:
  Sum/1 -> Sqrt/1
  x/1 -> Math Function1/1
  Sqrt/1 -> RMS/1
  Math Function1/1 -> Sum/1
  y/1 -> Math Function2/1
  Math Function2/1 -> Sum/2

== system SimplusGT/Single Pulse ==
  note: Pulse generator
      |
      | Author(s): Yitong Li
  Gain : Gain  Gain=Am
  Product : Product
  Step : Step  Time=t0  SampleTime=0
  Step1 : Step  Time=t0+dt  Before=1  After=0  SampleTime=0
  Out : Outport
  wires:
  Step1/1 -> Product/2
  Step/1 -> Product/1
  Product/1 -> Gain/1
  Gain/1 -> Out/1

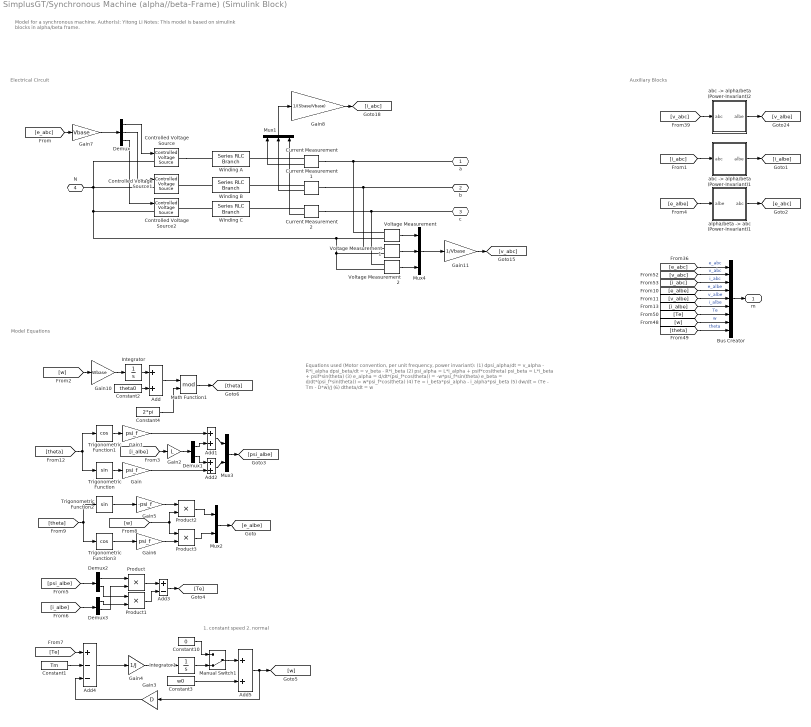
== system SimplusGT/Synchronous Machine (alpha//beta-Frame) (Simulink Block) ==
  note: 1. constant speed
      | 2. normal
  note: Auxiliary Blocks
  note: Model Equations
  note: Electrical Circuit
  note: Equations used
      | (Motor convention, per unit frequency, power invariant):
      |
      | (1) dpsi_alpha/dt = v_alpha - R*i_alpha
      | dpsi_beta/dt = v_beta - R*i_beta
      |
      | (2) psi_alpha = L*i_alpha + psif*cos(theta)
      | psi_beta = L*i_beta + psif*sin(theta)
      |
      | (3) e_alpha = d/dt*(psi_f*cos(theta)) = -w*psi_f*sin(theta)
      | e_beta = d/dt*(psi_f*sin(theta)) = w*psi_f*cos(theta)
      |
      | (4) Te = i_beta*psi_alpha - i_alpha*psi_beta
      | (5) dw/dt = (Te - Tm - D*w)/J
      | (6) dtheta/dt = w
  note: Model for a synchronous machine.
      |
      | Author(s): Yitong Li
      |
      | Notes:
      |
      | This model is based on simulink blocks in alpha/beta frame.
  Add{,1..2,5} (4 alike) : Sum
  Add3 : Sum  Inputs=+-
  Add4 : Sum  Inputs=+--
  Bus Creator : BusCreator  Inputs=9
  Constant1 : Constant  Value=Tm
  Constant10 : Constant  Value=0
  Constant2 : Constant  Value=theta0
  Constant3 : Constant  Value=w0
  Constant4 : Constant  Value=2*pi
  Controlled Voltage Source : powerlib/Electrical Sources/Controlled Voltage Source  Initialize=on  Source_Type=AC  Amplitude=0  Phase=0  Frequency=0  Measurements=None
  Controlled Voltage Source1 : powerlib/Electrical Sources/Controlled Voltage Source  Initialize=on  Source_Type=AC  Amplitude=0  Phase=0  Frequency=0  Measurements=None
  Controlled Voltage Source2 : powerlib/Electrical Sources/Controlled Voltage Source  Initialize=on  Source_Type=AC  Amplitude=0  Phase=0  Frequency=0  Measurements=None
  Current Measurement : powerlib/Measurements/Current Measurement  PhasorSimulation=off  OutputType=Complex  PSBequivalent=0
  Current Measurement1 : powerlib/Measurements/Current Measurement  PhasorSimulation=off  OutputType=Complex  PSBequivalent=0
  Current Measurement2 : powerlib/Measurements/Current Measurement  PhasorSimulation=off  OutputType=Complex  PSBequivalent=0
  Demux : Demux  Outputs=3
  Demux1 : Demux  Outputs=2
  Demux2 : Demux  Outputs=2
  Demux3 : Demux  Outputs=2
  Gain : Gain  Gain=psi_f
  Gain1 : Gain  Gain=psi_f
  Gain10 : Gain  Gain=Wbase
  Gain11 : Gain  Gain=1/Vbase
  Gain2 : Gain  Gain=L
  Gain3 : Gain  Gain=D
  Gain4 : Gain  Gain=1/J
  Gain5 : Gain  Gain=-psi_f
  Gain6 : Gain  Gain=psi_f
  Gain7 : Gain  Gain=Vbase
  Gain8 : Gain  Gain=1/(Sbase/Vbase)
  Integrator : Integrator
  Integrator1 : Integrator
  Manual Switch1 : ManualSwitch  CurrentSetting=0
  Math Function1 : Math  Operator=mod  SaturateOnIntegerOverflow=on
  Mux1 : Mux  Inputs=3
  Mux2 : Mux  Inputs=2
  Mux3 : Mux  Inputs=2
  Mux4 : Mux  Inputs=3
  Product{,1..3} (4 alike) : Product
  Trigonometric Function : Trigonometry
  Trigonometric Function1 : Trigonometry  Operator=cos
  Trigonometric Function2 : Trigonometry
  Trigonometric Function3 : Trigonometry  Operator=cos
  Voltage Measurement : powerlib/Measurements/Voltage Measurement  PhasorSimulation=off  OutputType=Complex  PSBequivalent=0
  Voltage Measurement1 : powerlib/Measurements/Voltage Measurement  PhasorSimulation=off  OutputType=Complex  PSBequivalent=0
  Voltage Measurement2 : powerlib/Measurements/Voltage Measurement  PhasorSimulation=off  OutputType=Complex  PSBequivalent=0
  Winding A : powerlib/Elements/Series RLC Branch  LConnTagsString=__new0  RConnTagsString=__new0  BranchType=RL  Resistance=R*(Vbase^2)/Sbase  Inductance=L*(Vbase^2)/Sbase/Wbase  SetiL0=off  InitialCurrent=ia0  Capacitance=1e-6  Setx0=off  InitialVoltage=0  Measurements=None
  Winding B : powerlib/Elements/Series RLC Branch  LConnTagsString=__new0  RConnTagsString=__new0  BranchType=RL  Resistance=R*(Vbase^2)/Sbase  Inductance=L*(Vbase^2)/Sbase/Wbase  SetiL0=off  InitialCurrent=ia0  Capacitance=1e-6  Setx0=off  InitialVoltage=0  Measurements=None
  Winding C : powerlib/Elements/Series RLC Branch  LConnTagsString=__new0  RConnTagsString=__new0  BranchType=RL  Resistance=R*(Vbase^2)/Sbase  Inductance=L*(Vbase^2)/Sbase/Wbase  SetiL0=off  InitialCurrent=ia0  Capacitance=1e-6  Setx0=off  InitialVoltage=0  Measurements=None
  "abc -> alpha/beta (Power-Invariant)1" : Subsystem  AncestorBlock=|
      | SimplusGT/abc -> alpha//beta
      | (Power-Invariant)
  "abc -> alpha/beta (Power-Invariant)2" : Subsystem  AncestorBlock=|
      | SimplusGT/abc -> alpha//beta
      | (Power-Invariant)
  "alpha/beta -> abc (Power-Invariant)1" : Subsystem  AncestorBlock=|
      | SimplusGT/alpha//beta -> abc
      | (Power-Invariant)
  a : PMIOPort  Side=Left
  b : PMIOPort  Port=2  Side=Left
  c : PMIOPort  Port=3  Side=Left
  N : PMIOPort  Port=4  Side=Left
  m : Outport
  wires:
  Current Measurement/1 -> Mux1/1
  Current Measurement1/1 -> Mux1/2
  Current Measurement2/1 -> Mux1/3
  Mux1/1 -> Gain8/1
  [e_abc] -> Gain7/1
  Demux/1 -> Controlled Voltage Source/1
  Demux/2 -> Controlled Voltage Source1/1
  Demux/3 -> Controlled Voltage Source2/1
  [i_abc] -> "abc -> alpha/beta (Power-Invariant)1"/1(abc)
  "abc -> alpha/beta (Power-Invariant)1"/1(albe) -> [i_albe]
  [w] -> Gain10/1
  Integrator/1 -> Add/1
  Constant2/1 -> Add/2
  Trigonometric Function1/1 -> Gain1/1
  Trigonometric Function/1 -> Gain/1
  [i_albe] -> Gain2/1
  Demux1/1 -> Add1/2
  Demux1/2 -> Add2/1
  Gain2/1 -> Demux1/1
  Gain1/1 -> Add1/1
  Gain/1 -> Add2/2
  Product2/1 -> Mux2/1
  Product3/1 -> Mux2/2
  Mux2/1 -> [e_albe]
  [e_albe] -> "alpha/beta -> abc (Power-Invariant)1"/1(albe)
  "alpha/beta -> abc (Power-Invariant)1"/1(abc) -> [e_abc]
  Add1/1 -> Mux3/1
  Add2/1 -> Mux3/2
  Mux3/1 -> [psi_albe]
  [psi_albe] -> Demux2/1
  [i_albe] -> Demux3/1
  Demux2/1 -> Product/1
  Demux3/2 -> Product/2
  Demux3/1 -> Product1/2
  Demux2/2 -> Product1/1
  Product/1 -> Add3/1
  Product1/1 -> Add3/2
  Add3/1 -> [Te]
  [Te] -> Add4/1
  Constant1/1 -> Add4/2
  Add4/1 -> Gain4/1
  Gain3/1 -> Add4/3
  Constant3/1 -> Add5/2
  Add5/1 -> Gain3/1, [w]
  [theta] -> Trigonometric Function3/1, Trigonometric Function2/1
  Trigonometric Function2/1 -> Gain5/1
  Trigonometric Function3/1 -> Gain6/1
  Gain5/1 -> Product2/1
  Gain6/1 -> Product3/2
  Gain8/1 -> [i_abc]
  Gain4/1 -> Integrator1/1
  Gain10/1 -> Integrator/1
  Voltage Measurement/1 -> Mux4/1
  Voltage Measurement1/1 -> Mux4/2
  Voltage Measurement2/1 -> Mux4/3
  Mux4/1 -> Gain11/1
  Gain11/1 -> [v_abc]
  Gain7/1 -> Demux/1
  Add/1 -> Math Function1/1
  Constant4/1 -> Math Function1/2
  Math Function1/1 -> [theta]
  [v_abc] -> "abc -> alpha/beta (Power-Invariant)2"/1(abc)
  "abc -> alpha/beta (Power-Invariant)2"/1(albe) -> [v_albe]
  [w] -> Product3/1, Product2/2
  [theta] -> Trigonometric Function/1, Trigonometric Function1/1
  Integrator1/1 -> Manual Switch1/2
  Manual Switch1/1 -> Add5/1
  Constant10/1 -> Manual Switch1/1
  [e_abc] -> Bus Creator/1  "e_abc"
  [v_abc] -> Bus Creator/2  "v_abc"
  [i_abc] -> Bus Creator/3  "i_abc"
  [e_albe] -> Bus Creator/4  "e_albe"
  [v_albe] -> Bus Creator/5  "v_albe"
  [i_albe] -> Bus Creator/6  "i_albe"
  [Te] -> Bus Creator/7  "Te"
  [w] -> Bus Creator/8  "w"
  [theta] -> Bus Creator/9  "theta"
  Bus Creator/1 -> m/1
  connections:
  Current Measurement/RConn1 -- Winding A/RConn1
  Controlled Voltage Source/RConn1 -- Winding A/LConn1
  Current Measurement2/RConn1 -- Winding C/RConn1
  Current Measurement/LConn1 -- Voltage Measurement/LConn1 -- a/RConn1
  Current Measurement1/LConn1 -- Voltage Measurement1/LConn1 -- b/RConn1
  Current Measurement1/RConn1 -- Winding B/RConn1
  Winding B/LConn1 -- Controlled Voltage Source1/RConn1
  Controlled Voltage Source/LConn1 -- Voltage Measurement2/LConn2 -- Voltage Measurement1/LConn2 -- Voltage Measurement/LConn2 -- Controlled Voltage Source2/LConn1 -- N/RConn1 -- Controlled Voltage Source1/LConn1
  Winding C/LConn1 -- Controlled Voltage Source2/RConn1
  Current Measurement2/LConn1 -- Voltage Measurement2/LConn1 -- c/RConn1
